simulink model "CarUncertaintyAnalysis"  (R2020b)
settings: Solver=VariableStepAuto  StartTime=0.0  StopTime=60  RelTol=1e-3
undefined symbols (not defined in the file): Area, Cri, CrN, Cv, delayi, F1, F2, FMax, g, H1, H2, mGrid, mi, rho, smi, tauActi, v0Grid, windAvei
libraries: simulink x3
settings Model: Creator=DELL  LastModifiedBy=DELL
settings SFSimCC: CustomCodeUndefinedFunction=UseInterfaceOnly

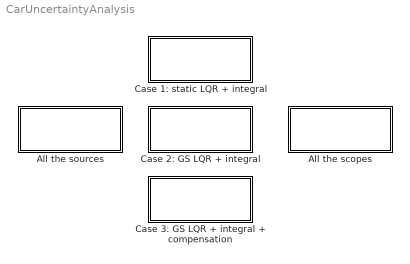
== system CarUncertaintyAnalysis ==
  All the scopes : Subsystem
  All the sources : Subsystem
  Case 1: static LQR + integral : Subsystem
  Case 2: GS LQR + integral : Subsystem
  Case 3: GS LQR + integral + compensation : Subsystem

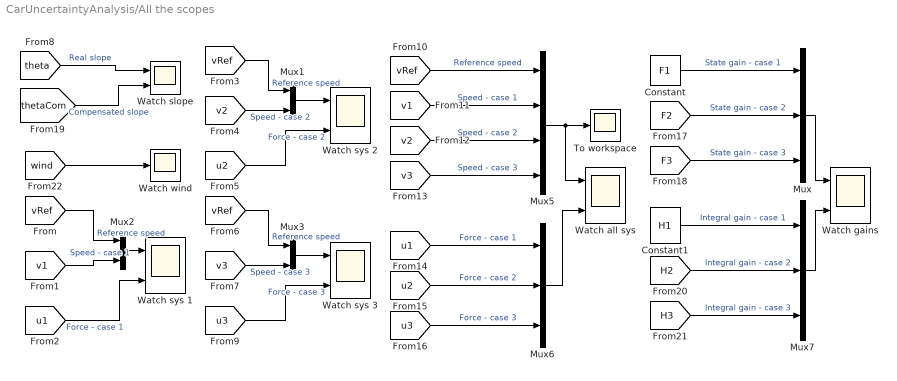
== system CarUncertaintyAnalysis/All the scopes ==
  Constant : Constant  Value=F1
  Constant1 : Constant  Value=H1
  Mux : Mux  Inputs=3
  Mux1 : Mux  Inputs=2
  Mux2 : Mux  Inputs=2
  Mux3 : Mux  Inputs=2
  Mux5 : Mux
  Mux6 : Mux  Inputs=3
  Mux7 : Mux  Inputs=3
  To workspace : Scope
  Watch all sys : Scope  NumInputPorts=2
  Watch gains : Scope  NumInputPorts=2
  Watch slope : Scope  NumInputPorts=2
  Watch sys 1 : Scope  NumInputPorts=2
  Watch sys 2 : Scope  NumInputPorts=2
  Watch sys 3 : Scope  NumInputPorts=2
  Watch wind : Scope
  wires:
  Mux/1 -> Watch gains/1
  Mux7/1 -> Watch gains/2
  Mux2/1 -> Watch sys 1/1
  [vRef] -> Mux2/1  "Reference speed"
  [u1] -> Watch sys 1/2  "Force - case 1"
  [v2] -> Mux1/2  "Speed - case 2"
  Mux1/1 -> Watch sys 2/1
  [vRef] -> Mux1/1  "Reference speed"
  [u2] -> Watch sys 2/2  "Force - case 2"
  [vRef] -> Mux3/1  "Reference speed"
  Mux3/1 -> Watch sys 3/1
  [v3] -> Mux3/2  "Speed - case 3"
  [u3] -> Watch sys 3/2  "Force - case 3"
  [v1] -> Mux2/2  "Speed - case 1"
  Mux5/1 -> To workspace/1, Watch all sys/1
  Mux6/1 -> Watch all sys/2
  [vRef] -> Mux5/1  "Reference speed"
  [v1] -> Mux5/2  "Speed - case 1"
  [v2] -> Mux5/3  "Speed - case 2"
  [v3] -> Mux5/4  "Speed - case 3"
  [u1] -> Mux6/1  "Force - case 1"
  [u2] -> Mux6/2  "Force - case 2"
  [u3] -> Mux6/3  "Force - case 3"
  Constant/1 -> Mux/1  "State gain - case 1"
  [F2] -> Mux/2  "State gain - case 2"
  [F3] -> Mux/3  "State gain - case 3"
  Constant1/1 -> Mux7/1  "Integral gain - case 1"
  [H2] -> Mux7/2  "Integral gain - case 2"
  [H3] -> Mux7/3  "Integral gain - case 3"
  [theta] -> Watch slope/1  "Real slope"
  [thetaCom] -> Watch slope/2  "Compensated slope"
  [wind] -> Watch wind/1

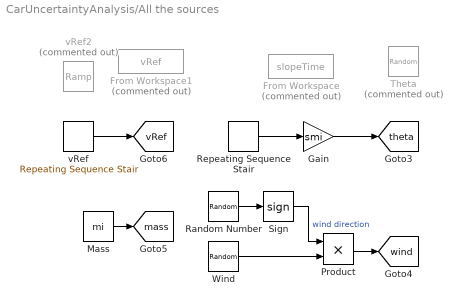
== system CarUncertaintyAnalysis/All the sources ==
  From Workspace : FromWorkspace  Commented=on  VariableName=slopeTime
  From Workspace1 : FromWorkspace  Commented=on  VariableName=vRef
  Gain : Gain  Gain=smi
  Mass : Constant  Value=mi
  Product : Product
  Random Number : RandomNumber  Variance=0.1  SampleTime=1
  Repeating Sequence Stair : simulink/Sources/Repeating Sequence Stair  OutValues=(pi/180)*[0 3 6 3 0 -3 -6 -3].'  tsamp=0.5  OutMin=[]  OutMax=[]  OutDataTypeStr=double  OutputDataTypeScalingMode=double  OutDataType=fixdt(0,8)  ConRadixGroup=Best Precision: Vector-wise  OutScaling=2^-12
  Sign : Signum
  Theta : RandomNumber  Commented=on  Variance=0.1  SampleTime=0.1
  Wind : RandomNumber  Mean=windAvei  Variance=10  SampleTime=1
  vRef : simulink/Sources/Repeating Sequence Stair  OutValues=[25 20].'  tsamp=10  OutMin=[]  OutMax=[]  OutDataTypeStr=double  OutputDataTypeScalingMode=double  OutDataType=fixdt(0,8)  ConRadixGroup=Best Precision: Vector-wise  OutScaling=2^-12
  vRef2 : simulink/Sources/Ramp  Commented=on  slope=0.5  start=0  InitialOutput=0
  tag scope: mass=global, theta=global, vRef=global, wind=global
  wires:
  vRef/1 -> [vRef]
  Mass/1 -> [mass]
  Random Number/1 -> Sign/1
  Wind/1 -> Product/2
  Sign/1 -> Product/1  "wind direction"
  Product/1 -> [wind]
  Gain/1 -> [theta]
  Repeating Sequence Stair/1 -> Gain/1

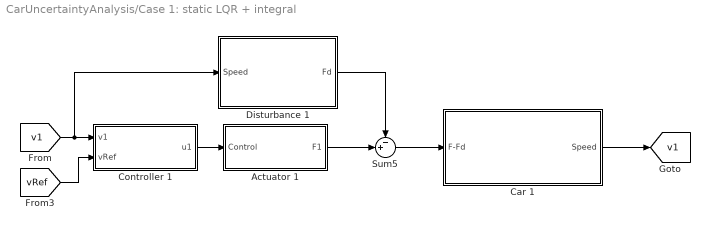
== system CarUncertaintyAnalysis/Case 1: static LQR + integral ==
  Actuator 1 : Subsystem
  Car 1 : Subsystem
  Controller 1 : Subsystem
  Disturbance 1 : Subsystem
  Sum5 : Sum  Inputs=-+|
  tag scope: v1=global
  wires:
  Controller 1/1(u1) -> Actuator 1/1(Control)
  Actuator 1/1(F1) -> Sum5/2
  Disturbance 1/1(Fd) -> Sum5/1
  [vRef] -> Controller 1/2(vRef)
  Sum5/1 -> Car 1/1("F-Fd ")
  Car 1/1(Speed) -> [v1]
  [v1] -> Disturbance 1/1(Speed), Controller 1/1(v1)

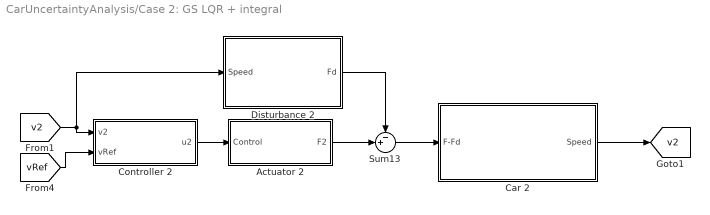
== system CarUncertaintyAnalysis/Case 2: GS LQR + integral ==
  Actuator 2 : Subsystem
  Car 2 : Subsystem
  Controller 2 : Subsystem
  Disturbance 2 : Subsystem
  Sum13 : Sum  Inputs=-+|
  tag scope: v2=global
  wires:
  Controller 2/1(u2) -> Actuator 2/1(Control)
  [vRef] -> Controller 2/2(vRef)
  Car 2/1(Speed) -> [v2]
  [v2] -> Disturbance 2/1(Speed), Controller 2/1(v2)
  Actuator 2/1(F2) -> Sum13/2
  Disturbance 2/1(Fd) -> Sum13/1
  Sum13/1 -> Car 2/1("F-Fd ")

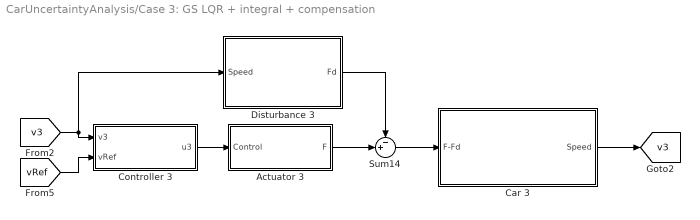
== system CarUncertaintyAnalysis/Case 3: GS LQR + integral + compensation ==
  Actuator 3 : Subsystem
  Car 3 : Subsystem
  Controller 3 : Subsystem
  Disturbance 3 : Subsystem
  Sum14 : Sum  Inputs=-+|
  tag scope: v3=global
  wires:
  Disturbance 3/1(Fd) -> Sum14/1
  Controller 3/1(u3) -> Actuator 3/1(Control)
  [vRef] -> Controller 3/2(vRef)
  [v3] -> Disturbance 3/1(Speed), Controller 3/1(v3)
  Actuator 3/1(F) -> Sum14/2
  Sum14/1 -> Car 3/1("F-Fd ")
  Car 3/1(Speed) -> [v3]

== system CarUncertaintyAnalysis/Case 1: static LQR + integral/Actuator 1 ==
  Control : Inport
  Actuator : TransferFcn  Denominator=[tauActi 1]
  Saturation : Saturate  UpperLimit=FMax  LowerLimit=-FMax
  Transport Delay1 : TransportDelay  DelayTime=delayi
  F1 : Outport  VectorParamsAs1DForOutWhenUnconnected=off
  tag scope: u1=global
  wires:
  Actuator/1 -> Saturation/1  "F"
  Saturation/1 -> Transport Delay1/1
  Control/1 -> Actuator/1
  Transport Delay1/1 -> [u1], F1/1

== system CarUncertaintyAnalysis/Case 1: static LQR + integral/Car 1 ==
  "F-Fd " : Inport
  Gain2 : Gain  Gain=1/mi
  Integrator1 : Integrator  InitialCondition=20
  Speed : Outport  VectorParamsAs1DForOutWhenUnconnected=off
  wires:
  Gain2/1 -> Integrator1/1  "v dot"
  "F-Fd "/1 -> Gain2/1  "F-Fd"
  Integrator1/1 -> Speed/1  "Speed"

== system CarUncertaintyAnalysis/Case 1: static LQR + integral/Controller 1 ==
  v1 : Inport
  vRef : Inport  Port=2
  Gain : Gain  Gain=F1
  Gain1 : Gain  Gain=H1
  Integrator : Integrator
  Sum : Sum  Inputs=|--
  Sum1 : Sum  Inputs=|+-
  u1 : Outport  VectorParamsAs1DForOutWhenUnconnected=off
  wires:
  Gain1/1 -> Sum/1
  Integrator/1 -> Gain1/1
  Gain/1 -> Sum/2
  Sum1/1 -> Integrator/1  "dv"
  Sum/1 -> u1/1
  vRef/1 -> Sum1/1
  v1/1 -> Sum1/2, Gain/1

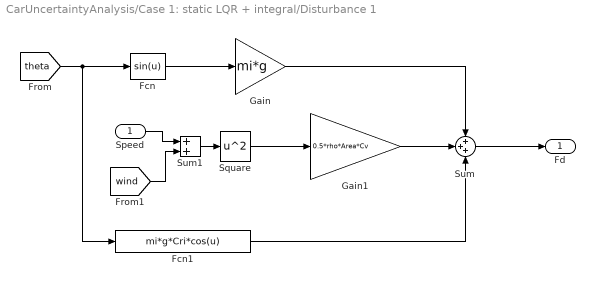
== system CarUncertaintyAnalysis/Case 1: static LQR + integral/Disturbance 1 ==
  Speed : Inport
  Fcn : Fcn  Expr=sin(u)
  Fcn1 : Fcn  Expr=mi*g*Cri*cos(u)
  Gain : Gain  Gain=mi*g
  Gain1 : Gain  Gain=0.5*rho*Area*Cv
  Square : Math  Operator=square  SignedPower=on  SaturateOnIntegerOverflow=on
  Sum : Sum  Inputs=+++
  Sum1 : Sum
  Fd : Outport  VectorParamsAs1DForOutWhenUnconnected=off
  wires:
  [theta] -> Fcn1/1, Fcn/1
  Square/1 -> Gain1/1
  Gain/1 -> Sum/1
  Gain1/1 -> Sum/2
  Fcn1/1 -> Sum/3
  Sum/1 -> Fd/1
  Fcn/1 -> Gain/1
  Sum1/1 -> Square/1
  Speed/1 -> Sum1/1
  [wind] -> Sum1/2

== system CarUncertaintyAnalysis/Case 2: GS LQR + integral/Actuator 2 ==
  Control : Inport
  Actuator : TransferFcn  Denominator=[tauActi 1]
  Saturation : Saturate  UpperLimit=FMax  LowerLimit=-FMax
  Transport Delay1 : TransportDelay  DelayTime=delayi
  F2 : Outport  VectorParamsAs1DForOutWhenUnconnected=off
  tag scope: u2=global
  wires:
  Control/1 -> Actuator/1
  Saturation/1 -> Transport Delay1/1
  Actuator/1 -> Saturation/1  "F"
  Transport Delay1/1 -> [u2], F2/1

== system CarUncertaintyAnalysis/Case 2: GS LQR + integral/Car 2 ==
  "F-Fd " : Inport
  Divide : Product  Inputs=*/
  Integrator1 : Integrator  InitialCondition=20
  Speed : Outport  VectorParamsAs1DForOutWhenUnconnected=off
  wires:
  Divide/1 -> Integrator1/1  "v dot"
  "F-Fd "/1 -> Divide/1  "F-Fd"
  Integrator1/1 -> Speed/1  "Speed"
  [mass] -> Divide/2

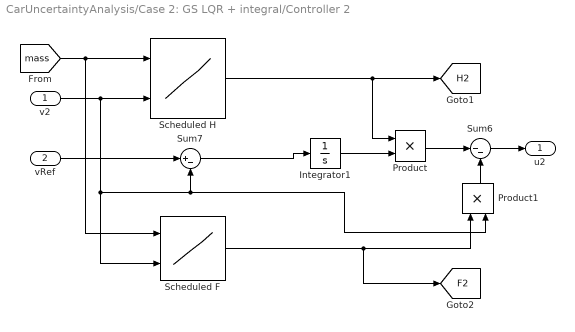
== system CarUncertaintyAnalysis/Case 2: GS LQR + integral/Controller 2 ==
  v2 : Inport
  vRef : Inport  Port=2
  Integrator1 : Integrator
  Product : Product
  Product1 : Product
  Scheduled F : Lookup_n-D  BreakpointsForDimension1=mGrid  BreakpointsForDimension2=v0Grid  Table=F2  InternalRulePriority=Speed  RndMeth=Simplest  InputSameDT=on
      settings: InputPortMap=u0,u1
  Scheduled H : Lookup_n-D  BreakpointsForDimension1=mGrid  BreakpointsForDimension2=v0Grid  Table=H2  InternalRulePriority=Speed  RndMeth=Simplest  InputSameDT=on
      settings: InputPortMap=u0,u1
  Sum6 : Sum  Inputs=|--
  Sum7 : Sum  Inputs=|+-
  u2 : Outport  VectorParamsAs1DForOutWhenUnconnected=off
  tag scope: F2=global, H2=global
  wires:
  Product/1 -> Sum6/1
  Product1/1 -> Sum6/2
  Sum7/1 -> Integrator1/1
  Scheduled F/1 -> [F2], Product1/1
  Scheduled H/1 -> [H2], Product/1
  Integrator1/1 -> Product/2
  [mass] -> Scheduled F/1, Scheduled H/1
  vRef/1 -> Sum7/1
  Sum6/1 -> u2/1
  v2/1 -> Scheduled F/2, Sum7/2, Product1/2, Scheduled H/2

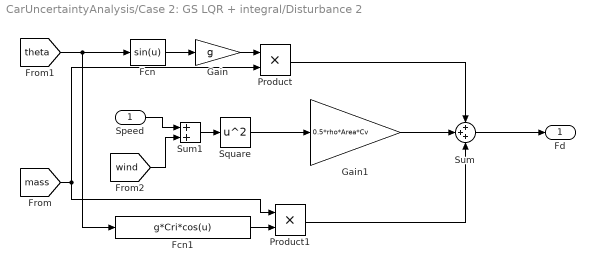
== system CarUncertaintyAnalysis/Case 2: GS LQR + integral/Disturbance 2 ==
  Speed : Inport
  Fcn : Fcn  Expr=sin(u)
  Fcn1 : Fcn  Expr=g*Cri*cos(u)
  Gain : Gain  Gain=g
  Gain1 : Gain  Gain=0.5*rho*Area*Cv
  Product : Product
  Product1 : Product
  Square : Math  Operator=square  SignedPower=on  SaturateOnIntegerOverflow=on
  Sum : Sum  Inputs=+++
  Sum1 : Sum
  Fd : Outport  VectorParamsAs1DForOutWhenUnconnected=off
  wires:
  [theta] -> Fcn1/1, Fcn/1
  Square/1 -> Gain1/1
  Gain1/1 -> Sum/2
  Sum/1 -> Fd/1
  Fcn/1 -> Gain/1
  Sum1/1 -> Square/1
  Speed/1 -> Sum1/1
  Product/1 -> Sum/1
  Gain/1 -> Product/1
  [mass] -> Product1/1, Product/2
  Fcn1/1 -> Product1/2
  Product1/1 -> Sum/3
  [wind] -> Sum1/2

== system CarUncertaintyAnalysis/Case 3: GS LQR + integral + compensation/Actuator 3 ==
  Control : Inport
  Actuator : TransferFcn  Denominator=[tauActi 1]
  Saturation : Saturate  UpperLimit=FMax  LowerLimit=-FMax
  Transport Delay1 : TransportDelay  DelayTime=delayi
  F : Outport  VectorParamsAs1DForOutWhenUnconnected=off
  tag scope: u3=global
  wires:
  Control/1 -> Actuator/1
  Saturation/1 -> Transport Delay1/1
  Actuator/1 -> Saturation/1  "F"
  Transport Delay1/1 -> [u3], F/1

== system CarUncertaintyAnalysis/Case 3: GS LQR + integral + compensation/Car 3 ==
  "F-Fd " : Inport
  Divide : Product  Inputs=*/
  Integrator1 : Integrator  InitialCondition=20
  Speed : Outport  VectorParamsAs1DForOutWhenUnconnected=off
  wires:
  Divide/1 -> Integrator1/1  "v dot"
  "F-Fd "/1 -> Divide/1  "F-Fd"
  Integrator1/1 -> Speed/1  "Speed"
  [mass] -> Divide/2

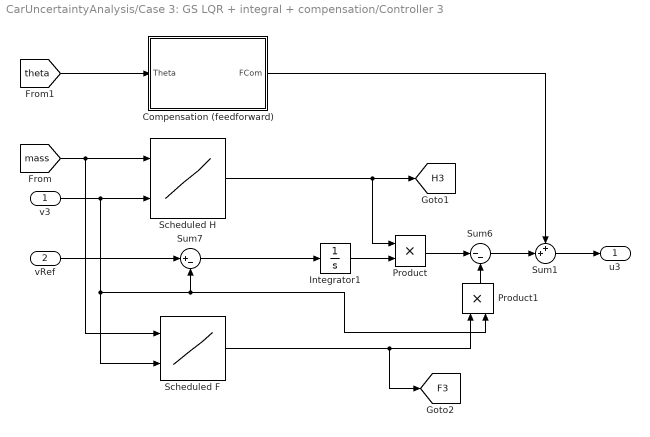
== system CarUncertaintyAnalysis/Case 3: GS LQR + integral + compensation/Controller 3 ==
  v3 : Inport
  vRef : Inport  Port=2
  "Compensation (feedforward) " : Subsystem
  Integrator1 : Integrator
  Product : Product
  Product1 : Product
  Scheduled F : Lookup_n-D  BreakpointsForDimension1=mGrid  BreakpointsForDimension2=v0Grid  Table=F2  InternalRulePriority=Speed  RndMeth=Simplest  InputSameDT=on
      settings: InputPortMap=u0,u1
  Scheduled H : Lookup_n-D  BreakpointsForDimension1=mGrid  BreakpointsForDimension2=v0Grid  Table=H2  InternalRulePriority=Speed  RndMeth=Simplest  InputSameDT=on
      settings: InputPortMap=u0,u1
  Sum1 : Sum  Inputs=++|
  Sum6 : Sum  Inputs=|--
  Sum7 : Sum  Inputs=|+-
  u3 : Outport  VectorParamsAs1DForOutWhenUnconnected=off
  tag scope: F3=global, H3=global
  wires:
  v3/1 -> Scheduled H/2, Scheduled F/2, Sum7/2, Product1/2
  [mass] -> Scheduled F/1, Scheduled H/1
  vRef/1 -> Sum7/1
  Integrator1/1 -> Product/2
  Sum7/1 -> Integrator1/1
  Scheduled F/1 -> [F3], Product1/1
  Product1/1 -> Sum6/2
  Product/1 -> Sum6/1
  Sum1/1 -> u3/1
  Sum6/1 -> Sum1/2
  "Compensation (feedforward) "/1(FCom) -> Sum1/1
  [theta] -> "Compensation (feedforward) "/1(Theta)
  Scheduled H/1 -> [H3], Product/1

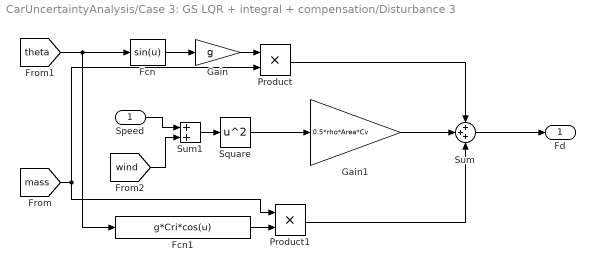
== system CarUncertaintyAnalysis/Case 3: GS LQR + integral + compensation/Disturbance 3 ==
  Speed : Inport
  Fcn : Fcn  Expr=sin(u)
  Fcn1 : Fcn  Expr=g*Cri*cos(u)
  Gain : Gain  Gain=g
  Gain1 : Gain  Gain=0.5*rho*Area*Cv
  Product : Product
  Product1 : Product
  Square : Math  Operator=square  SignedPower=on  SaturateOnIntegerOverflow=on
  Sum : Sum  Inputs=+++
  Sum1 : Sum
  Fd : Outport  VectorParamsAs1DForOutWhenUnconnected=off
  wires:
  [wind] -> Sum1/2
  Product1/1 -> Sum/3
  Fcn1/1 -> Product1/2
  [mass] -> Product/2, Product1/1
  Gain/1 -> Product/1
  Product/1 -> Sum/1
  Speed/1 -> Sum1/1
  Sum1/1 -> Square/1
  Fcn/1 -> Gain/1
  Sum/1 -> Fd/1
  Gain1/1 -> Sum/2
  Square/1 -> Gain1/1
  [theta] -> Fcn/1, Fcn1/1

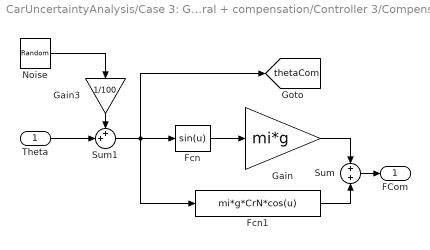
== system CarUncertaintyAnalysis/Case 3: GS LQR + integral + compensation/Controller 3/Compensation (feedforward)  ==
  Theta : Inport
  Fcn : Fcn  Expr=sin(u)
  Fcn1 : Fcn  Expr=mi*g*CrN*cos(u)
  Gain : Gain  Gain=mi*g
  Gain3 : Gain  Gain=1/100
  Noise : RandomNumber  Variance=10  SampleTime=0.1
  Sum : Sum  Inputs=+|+
  Sum1 : Sum  Inputs=++|
  FCom : Outport  VectorParamsAs1DForOutWhenUnconnected=off
  tag scope: thetaCom=global
  wires:
  Gain/1 -> Sum/1
  Fcn1/1 -> Sum/2
  Fcn/1 -> Gain/1
  Sum/1 -> FCom/1
  Noise/1 -> Gain3/1
  Gain3/1 -> Sum1/1
  Theta/1 -> Sum1/2
  Sum1/1 -> [thetaCom], Fcn1/1, Fcn/1
